simulink model "c00019M_harness"  (R2018a)
settings: Solver=ode3  StartTime=0.0  StopTime=10.0  RelTol=1e-3  EnableMultiTasking=on
undefined symbols (not defined in the file): b, DiscIntNeverNeededParam, J, K, L, PosMinimaW4, R, sigbuilder_block
(part 3 of 43)

== system c00019M_harness/Eval14 ==
  In1 : Inport
  In2 : Inport  Port=2
  In4 : Inport  Port=3
  Constant3 : Constant
  Data Type Conversion : DataTypeConversion
  Data Type Conversion1 : DataTypeConversion
  Data Type Conversion3 : DataTypeConversion
  Memory1 : Memory  InitialCondition=1
  Memory2 : Memory  InitialCondition=1
  Memory4 : Memory  InitialCondition=1
  MinMax : MinMax  Inputs=4
  MinMax1 : MinMax  Inputs=2
  MinMax2 : MinMax  Inputs=2
  MinMax4 : MinMax  Inputs=2
  ROOut1 : RelationalOperator  Operator===  OutDataTypeStr=boolean  RndMeth=Simplest
  ROOut2 : RelationalOperator  Operator===  OutDataTypeStr=boolean  RndMeth=Simplest
  ROOut4 : RelationalOperator  Operator===  OutDataTypeStr=boolean  RndMeth=Simplest
  Out1 : Outport
  wires:
  Data Type Conversion3/1 -> MinMax4/1
  Data Type Conversion1/1 -> MinMax2/1
  Data Type Conversion/1 -> MinMax1/1
  MinMax1/1 -> Memory1/1, MinMax/1
  ROOut4/1 -> Data Type Conversion3/1
  MinMax2/1 -> Memory2/1, MinMax/2
  ROOut1/1 -> Data Type Conversion/1
  Memory2/1 -> MinMax2/2
  Memory4/1 -> MinMax4/2
  ROOut2/1 -> Data Type Conversion1/1
  MinMax4/1 -> Memory4/1, MinMax/4
  Memory1/1 -> MinMax1/2
  [out4] -> ROOut4/2
  In4/1 -> ROOut4/1
  [out2] -> ROOut2/2
  In1/1 -> ROOut1/1
  In2/1 -> ROOut2/1
  [out1] -> ROOut1/2
  MinMax/1 -> Out1/1
  Constant3/1 -> MinMax/3

== system c00019M_harness/Eval141 ==
  In1 : Inport
  In2 : Inport  Port=2
  In4 : Inport  Port=3
  Constant3 : Constant
  Data Type Conversion : DataTypeConversion
  Data Type Conversion1 : DataTypeConversion
  Data Type Conversion3 : DataTypeConversion
  Memory1 : Memory  InitialCondition=1
  Memory2 : Memory  InitialCondition=1
  Memory4 : Memory  InitialCondition=1
  MinMax : MinMax  Inputs=4
  MinMax1 : MinMax  Inputs=2
  MinMax2 : MinMax  Inputs=2
  MinMax4 : MinMax  Inputs=2
  ROOut1 : RelationalOperator  Operator===  OutDataTypeStr=boolean  RndMeth=Simplest
  ROOut2 : RelationalOperator  Operator===  OutDataTypeStr=boolean  RndMeth=Simplest
  ROOut4 : RelationalOperator  Operator===  OutDataTypeStr=boolean  RndMeth=Simplest
  Out1 : Outport
  wires:
  Data Type Conversion3/1 -> MinMax4/1
  Data Type Conversion1/1 -> MinMax2/1
  Data Type Conversion/1 -> MinMax1/1
  MinMax1/1 -> Memory1/1, MinMax/1
  ROOut4/1 -> Data Type Conversion3/1
  MinMax2/1 -> Memory2/1, MinMax/2
  ROOut1/1 -> Data Type Conversion/1
  Memory2/1 -> MinMax2/2
  Memory4/1 -> MinMax4/2
  ROOut2/1 -> Data Type Conversion1/1
  MinMax4/1 -> Memory4/1, MinMax/4
  Memory1/1 -> MinMax1/2
  [out4] -> ROOut4/2
  In4/1 -> ROOut4/1
  [out2] -> ROOut2/2
  In1/1 -> ROOut1/1
  In2/1 -> ROOut2/1
  [out1] -> ROOut1/2
  MinMax/1 -> Out1/1
  Constant3/1 -> MinMax/3

== system c00019M_harness/Eval142 ==
  In1 : Inport
  In2 : Inport  Port=2
  In4 : Inport  Port=3
  Constant3 : Constant
  Data Type Conversion : DataTypeConversion
  Data Type Conversion1 : DataTypeConversion
  Data Type Conversion3 : DataTypeConversion
  Memory1 : Memory  InitialCondition=1
  Memory2 : Memory  InitialCondition=1
  Memory4 : Memory  InitialCondition=1
  MinMax : MinMax  Inputs=4
  MinMax1 : MinMax  Inputs=2
  MinMax2 : MinMax  Inputs=2
  MinMax4 : MinMax  Inputs=2
  ROOut1 : RelationalOperator  Operator===  OutDataTypeStr=boolean  RndMeth=Simplest
  ROOut2 : RelationalOperator  Operator===  OutDataTypeStr=boolean  RndMeth=Simplest
  ROOut4 : RelationalOperator  Operator===  OutDataTypeStr=boolean  RndMeth=Simplest
  Out1 : Outport
  wires:
  Data Type Conversion3/1 -> MinMax4/1
  Data Type Conversion1/1 -> MinMax2/1
  Data Type Conversion/1 -> MinMax1/1
  MinMax1/1 -> Memory1/1, MinMax/1
  ROOut4/1 -> Data Type Conversion3/1
  MinMax2/1 -> Memory2/1, MinMax/2
  ROOut1/1 -> Data Type Conversion/1
  Memory2/1 -> MinMax2/2
  Memory4/1 -> MinMax4/2
  ROOut2/1 -> Data Type Conversion1/1
  MinMax4/1 -> Memory4/1, MinMax/4
  Memory1/1 -> MinMax1/2
  [out4] -> ROOut4/2
  In4/1 -> ROOut4/1
  [out2] -> ROOut2/2
  In1/1 -> ROOut1/1
  In2/1 -> ROOut2/1
  [out1] -> ROOut1/2
  MinMax/1 -> Out1/1
  Constant3/1 -> MinMax/3

== system c00019M_harness/Eval143 ==
  In1 : Inport
  In2 : Inport  Port=2
  In4 : Inport  Port=3
  Constant3 : Constant
  Data Type Conversion : DataTypeConversion
  Data Type Conversion1 : DataTypeConversion
  Data Type Conversion3 : DataTypeConversion
  Memory1 : Memory  InitialCondition=1
  Memory2 : Memory  InitialCondition=1
  Memory4 : Memory  InitialCondition=1
  MinMax : MinMax  Inputs=4
  MinMax1 : MinMax  Inputs=2
  MinMax2 : MinMax  Inputs=2
  MinMax4 : MinMax  Inputs=2
  ROOut1 : RelationalOperator  Operator===  OutDataTypeStr=boolean  RndMeth=Simplest
  ROOut2 : RelationalOperator  Operator===  OutDataTypeStr=boolean  RndMeth=Simplest
  ROOut4 : RelationalOperator  Operator===  OutDataTypeStr=boolean  RndMeth=Simplest
  Out1 : Outport
  wires:
  Data Type Conversion3/1 -> MinMax4/1
  Data Type Conversion1/1 -> MinMax2/1
  Data Type Conversion/1 -> MinMax1/1
  MinMax1/1 -> Memory1/1, MinMax/1
  ROOut4/1 -> Data Type Conversion3/1
  MinMax2/1 -> Memory2/1, MinMax/2
  ROOut1/1 -> Data Type Conversion/1
  Memory2/1 -> MinMax2/2
  Memory4/1 -> MinMax4/2
  ROOut2/1 -> Data Type Conversion1/1
  MinMax4/1 -> Memory4/1, MinMax/4
  Memory1/1 -> MinMax1/2
  [out4] -> ROOut4/2
  In4/1 -> ROOut4/1
  [out2] -> ROOut2/2
  In1/1 -> ROOut1/1
  In2/1 -> ROOut2/1
  [out1] -> ROOut1/2
  MinMax/1 -> Out1/1
  Constant3/1 -> MinMax/3

== system c00019M_harness/Eval145 ==
  In1 : Inport
  In2 : Inport  Port=2
  In4 : Inport  Port=3
  Constant3 : Constant
  Data Type Conversion : DataTypeConversion
  Data Type Conversion1 : DataTypeConversion
  Data Type Conversion3 : DataTypeConversion
  Memory1 : Memory  InitialCondition=1
  Memory2 : Memory  InitialCondition=1
  Memory4 : Memory  InitialCondition=1
  MinMax : MinMax  Inputs=4
  MinMax1 : MinMax  Inputs=2
  MinMax2 : MinMax  Inputs=2
  MinMax4 : MinMax  Inputs=2
  ROOut1 : RelationalOperator  Operator===  OutDataTypeStr=boolean  RndMeth=Simplest
  ROOut2 : RelationalOperator  Operator===  OutDataTypeStr=boolean  RndMeth=Simplest
  ROOut4 : RelationalOperator  Operator===  OutDataTypeStr=boolean  RndMeth=Simplest
  Out1 : Outport
  wires:
  Data Type Conversion3/1 -> MinMax4/1
  Data Type Conversion1/1 -> MinMax2/1
  Data Type Conversion/1 -> MinMax1/1
  MinMax1/1 -> Memory1/1, MinMax/1
  ROOut4/1 -> Data Type Conversion3/1
  MinMax2/1 -> Memory2/1, MinMax/2
  ROOut1/1 -> Data Type Conversion/1
  Memory2/1 -> MinMax2/2
  Memory4/1 -> MinMax4/2
  ROOut2/1 -> Data Type Conversion1/1
  MinMax4/1 -> Memory4/1, MinMax/4
  Memory1/1 -> MinMax1/2
  [out4] -> ROOut4/2
  In4/1 -> ROOut4/1
  [out2] -> ROOut2/2
  In1/1 -> ROOut1/1
  In2/1 -> ROOut2/1
  [out1] -> ROOut1/2
  MinMax/1 -> Out1/1
  Constant3/1 -> MinMax/3

== system c00019M_harness/Eval146 ==
  In1 : Inport
  In2 : Inport  Port=2
  In4 : Inport  Port=3
  Constant3 : Constant
  Data Type Conversion : DataTypeConversion
  Data Type Conversion1 : DataTypeConversion
  Data Type Conversion3 : DataTypeConversion
  Memory1 : Memory  InitialCondition=1
  Memory2 : Memory  InitialCondition=1
  Memory4 : Memory  InitialCondition=1
  MinMax : MinMax  Inputs=4
  MinMax1 : MinMax  Inputs=2
  MinMax2 : MinMax  Inputs=2
  MinMax4 : MinMax  Inputs=2
  ROOut1 : RelationalOperator  Operator===  OutDataTypeStr=boolean  RndMeth=Simplest
  ROOut2 : RelationalOperator  Operator===  OutDataTypeStr=boolean  RndMeth=Simplest
  ROOut4 : RelationalOperator  Operator===  OutDataTypeStr=boolean  RndMeth=Simplest
  Out1 : Outport
  wires:
  Data Type Conversion3/1 -> MinMax4/1
  Data Type Conversion1/1 -> MinMax2/1
  Data Type Conversion/1 -> MinMax1/1
  MinMax1/1 -> Memory1/1, MinMax/1
  ROOut4/1 -> Data Type Conversion3/1
  MinMax2/1 -> Memory2/1, MinMax/2
  ROOut1/1 -> Data Type Conversion/1
  Memory2/1 -> MinMax2/2
  Memory4/1 -> MinMax4/2
  ROOut2/1 -> Data Type Conversion1/1
  MinMax4/1 -> Memory4/1, MinMax/4
  Memory1/1 -> MinMax1/2
  [out4] -> ROOut4/2
  In4/1 -> ROOut4/1
  [out2] -> ROOut2/2
  In1/1 -> ROOut1/1
  In2/1 -> ROOut2/1
  [out1] -> ROOut1/2
  MinMax/1 -> Out1/1
  Constant3/1 -> MinMax/3

== system c00019M_harness/Eval147 ==
  In1 : Inport
  In2 : Inport  Port=2
  In4 : Inport  Port=3
  Constant3 : Constant
  Data Type Conversion : DataTypeConversion
  Data Type Conversion1 : DataTypeConversion
  Data Type Conversion3 : DataTypeConversion
  Memory1 : Memory  InitialCondition=1
  Memory2 : Memory  InitialCondition=1
  Memory4 : Memory  InitialCondition=1
  MinMax : MinMax  Inputs=4
  MinMax1 : MinMax  Inputs=2
  MinMax2 : MinMax  Inputs=2
  MinMax4 : MinMax  Inputs=2
  ROOut1 : RelationalOperator  Operator===  OutDataTypeStr=boolean  RndMeth=Simplest
  ROOut2 : RelationalOperator  Operator===  OutDataTypeStr=boolean  RndMeth=Simplest
  ROOut4 : RelationalOperator  Operator===  OutDataTypeStr=boolean  RndMeth=Simplest
  Out1 : Outport
  wires:
  Data Type Conversion3/1 -> MinMax4/1
  Data Type Conversion1/1 -> MinMax2/1
  Data Type Conversion/1 -> MinMax1/1
  MinMax1/1 -> Memory1/1, MinMax/1
  ROOut4/1 -> Data Type Conversion3/1
  MinMax2/1 -> Memory2/1, MinMax/2
  ROOut1/1 -> Data Type Conversion/1
  Memory2/1 -> MinMax2/2
  Memory4/1 -> MinMax4/2
  ROOut2/1 -> Data Type Conversion1/1
  MinMax4/1 -> Memory4/1, MinMax/4
  Memory1/1 -> MinMax1/2
  [out4] -> ROOut4/2
  In4/1 -> ROOut4/1
  [out2] -> ROOut2/2
  In1/1 -> ROOut1/1
  In2/1 -> ROOut2/1
  [out1] -> ROOut1/2
  MinMax/1 -> Out1/1
  Constant3/1 -> MinMax/3

== system c00019M_harness/Eval149 ==
  In1 : Inport
  In2 : Inport  Port=2
  In4 : Inport  Port=3
  Constant3 : Constant
  Data Type Conversion : DataTypeConversion
  Data Type Conversion1 : DataTypeConversion
  Data Type Conversion3 : DataTypeConversion
  Memory1 : Memory  InitialCondition=1
  Memory2 : Memory  InitialCondition=1
  Memory4 : Memory  InitialCondition=1
  MinMax : MinMax  Inputs=4
  MinMax1 : MinMax  Inputs=2
  MinMax2 : MinMax  Inputs=2
  MinMax4 : MinMax  Inputs=2
  ROOut1 : RelationalOperator  Operator===  OutDataTypeStr=boolean  RndMeth=Simplest
  ROOut2 : RelationalOperator  Operator===  OutDataTypeStr=boolean  RndMeth=Simplest
  ROOut4 : RelationalOperator  Operator===  OutDataTypeStr=boolean  RndMeth=Simplest
  Out1 : Outport
  wires:
  Data Type Conversion3/1 -> MinMax4/1
  Data Type Conversion1/1 -> MinMax2/1
  Data Type Conversion/1 -> MinMax1/1
  MinMax1/1 -> Memory1/1, MinMax/1
  ROOut4/1 -> Data Type Conversion3/1
  MinMax2/1 -> Memory2/1, MinMax/2
  ROOut1/1 -> Data Type Conversion/1
  Memory2/1 -> MinMax2/2
  Memory4/1 -> MinMax4/2
  ROOut2/1 -> Data Type Conversion1/1
  MinMax4/1 -> Memory4/1, MinMax/4
  Memory1/1 -> MinMax1/2
  [out4] -> ROOut4/2
  In4/1 -> ROOut4/1
  [out2] -> ROOut2/2
  In1/1 -> ROOut1/1
  In2/1 -> ROOut2/1
  [out1] -> ROOut1/2
  MinMax/1 -> Out1/1
  Constant3/1 -> MinMax/3

== system c00019M_harness/Eval15 ==
  In1 : Inport
  In2 : Inport  Port=2
  In4 : Inport  Port=3
  Constant3 : Constant
  Data Type Conversion : DataTypeConversion
  Data Type Conversion1 : DataTypeConversion
  Data Type Conversion3 : DataTypeConversion
  Memory1 : Memory  InitialCondition=1
  Memory2 : Memory  InitialCondition=1
  Memory4 : Memory  InitialCondition=1
  MinMax : MinMax  Inputs=4
  MinMax1 : MinMax  Inputs=2
  MinMax2 : MinMax  Inputs=2
  MinMax4 : MinMax  Inputs=2
  ROOut1 : RelationalOperator  Operator===  OutDataTypeStr=boolean  RndMeth=Simplest
  ROOut2 : RelationalOperator  Operator===  OutDataTypeStr=boolean  RndMeth=Simplest
  ROOut4 : RelationalOperator  Operator===  OutDataTypeStr=boolean  RndMeth=Simplest
  Out1 : Outport
  wires:
  Data Type Conversion3/1 -> MinMax4/1
  Data Type Conversion1/1 -> MinMax2/1
  Data Type Conversion/1 -> MinMax1/1
  MinMax1/1 -> Memory1/1, MinMax/1
  ROOut4/1 -> Data Type Conversion3/1
  MinMax2/1 -> Memory2/1, MinMax/2
  ROOut1/1 -> Data Type Conversion/1
  Memory2/1 -> MinMax2/2
  Memory4/1 -> MinMax4/2
  ROOut2/1 -> Data Type Conversion1/1
  MinMax4/1 -> Memory4/1, MinMax/4
  Memory1/1 -> MinMax1/2
  [out4] -> ROOut4/2
  In4/1 -> ROOut4/1
  [out2] -> ROOut2/2
  In1/1 -> ROOut1/1
  In2/1 -> ROOut2/1
  [out1] -> ROOut1/2
  MinMax/1 -> Out1/1
  Constant3/1 -> MinMax/3

== system c00019M_harness/Eval150 ==
  In1 : Inport
  In2 : Inport  Port=2
  In4 : Inport  Port=3
  Constant3 : Constant
  Data Type Conversion : DataTypeConversion
  Data Type Conversion1 : DataTypeConversion
  Data Type Conversion3 : DataTypeConversion
  Memory1 : Memory  InitialCondition=1
  Memory2 : Memory  InitialCondition=1
  Memory4 : Memory  InitialCondition=1
  MinMax : MinMax  Inputs=4
  MinMax1 : MinMax  Inputs=2
  MinMax2 : MinMax  Inputs=2
  MinMax4 : MinMax  Inputs=2
  ROOut1 : RelationalOperator  Operator===  OutDataTypeStr=boolean  RndMeth=Simplest
  ROOut2 : RelationalOperator  Operator===  OutDataTypeStr=boolean  RndMeth=Simplest
  ROOut4 : RelationalOperator  Operator===  OutDataTypeStr=boolean  RndMeth=Simplest
  Out1 : Outport
  wires:
  Data Type Conversion3/1 -> MinMax4/1
  Data Type Conversion1/1 -> MinMax2/1
  Data Type Conversion/1 -> MinMax1/1
  MinMax1/1 -> Memory1/1, MinMax/1
  ROOut4/1 -> Data Type Conversion3/1
  MinMax2/1 -> Memory2/1, MinMax/2
  ROOut1/1 -> Data Type Conversion/1
  Memory2/1 -> MinMax2/2
  Memory4/1 -> MinMax4/2
  ROOut2/1 -> Data Type Conversion1/1
  MinMax4/1 -> Memory4/1, MinMax/4
  Memory1/1 -> MinMax1/2
  [out4] -> ROOut4/2
  In4/1 -> ROOut4/1
  [out2] -> ROOut2/2
  In1/1 -> ROOut1/1
  In2/1 -> ROOut2/1
  [out1] -> ROOut1/2
  MinMax/1 -> Out1/1
  Constant3/1 -> MinMax/3

== system c00019M_harness/Eval151 ==
  In1 : Inport
  In2 : Inport  Port=2
  In4 : Inport  Port=3
  Constant3 : Constant
  Data Type Conversion : DataTypeConversion
  Data Type Conversion1 : DataTypeConversion
  Data Type Conversion3 : DataTypeConversion
  Memory1 : Memory  InitialCondition=1
  Memory2 : Memory  InitialCondition=1
  Memory4 : Memory  InitialCondition=1
  MinMax : MinMax  Inputs=4
  MinMax1 : MinMax  Inputs=2
  MinMax2 : MinMax  Inputs=2
  MinMax4 : MinMax  Inputs=2
  ROOut1 : RelationalOperator  Operator===  OutDataTypeStr=boolean  RndMeth=Simplest
  ROOut2 : RelationalOperator  Operator===  OutDataTypeStr=boolean  RndMeth=Simplest
  ROOut4 : RelationalOperator  Operator===  OutDataTypeStr=boolean  RndMeth=Simplest
  Out1 : Outport
  wires:
  Data Type Conversion3/1 -> MinMax4/1
  Data Type Conversion1/1 -> MinMax2/1
  Data Type Conversion/1 -> MinMax1/1
  MinMax1/1 -> Memory1/1, MinMax/1
  ROOut4/1 -> Data Type Conversion3/1
  MinMax2/1 -> Memory2/1, MinMax/2
  ROOut1/1 -> Data Type Conversion/1
  Memory2/1 -> MinMax2/2
  Memory4/1 -> MinMax4/2
  ROOut2/1 -> Data Type Conversion1/1
  MinMax4/1 -> Memory4/1, MinMax/4
  Memory1/1 -> MinMax1/2
  [out4] -> ROOut4/2
  In4/1 -> ROOut4/1
  [out2] -> ROOut2/2
  In1/1 -> ROOut1/1
  In2/1 -> ROOut2/1
  [out1] -> ROOut1/2
  MinMax/1 -> Out1/1
  Constant3/1 -> MinMax/3

== system c00019M_harness/Eval153 ==
  In1 : Inport
  In2 : Inport  Port=2
  In4 : Inport  Port=3
  Constant3 : Constant
  Data Type Conversion : DataTypeConversion
  Data Type Conversion1 : DataTypeConversion
  Data Type Conversion3 : DataTypeConversion
  Memory1 : Memory  InitialCondition=1
  Memory2 : Memory  InitialCondition=1
  Memory4 : Memory  InitialCondition=1
  MinMax : MinMax  Inputs=4
  MinMax1 : MinMax  Inputs=2
  MinMax2 : MinMax  Inputs=2
  MinMax4 : MinMax  Inputs=2
  ROOut1 : RelationalOperator  Operator===  OutDataTypeStr=boolean  RndMeth=Simplest
  ROOut2 : RelationalOperator  Operator===  OutDataTypeStr=boolean  RndMeth=Simplest
  ROOut4 : RelationalOperator  Operator===  OutDataTypeStr=boolean  RndMeth=Simplest
  Out1 : Outport
  wires:
  Data Type Conversion3/1 -> MinMax4/1
  Data Type Conversion1/1 -> MinMax2/1
  Data Type Conversion/1 -> MinMax1/1
  MinMax1/1 -> Memory1/1, MinMax/1
  ROOut4/1 -> Data Type Conversion3/1
  MinMax2/1 -> Memory2/1, MinMax/2
  ROOut1/1 -> Data Type Conversion/1
  Memory2/1 -> MinMax2/2
  Memory4/1 -> MinMax4/2
  ROOut2/1 -> Data Type Conversion1/1
  MinMax4/1 -> Memory4/1, MinMax/4
  Memory1/1 -> MinMax1/2
  [out4] -> ROOut4/2
  In4/1 -> ROOut4/1
  [out2] -> ROOut2/2
  In1/1 -> ROOut1/1
  In2/1 -> ROOut2/1
  [out1] -> ROOut1/2
  MinMax/1 -> Out1/1
  Constant3/1 -> MinMax/3

== system c00019M_harness/Eval154 ==
  In1 : Inport
  In2 : Inport  Port=2
  In4 : Inport  Port=3
  Constant3 : Constant
  Data Type Conversion : DataTypeConversion
  Data Type Conversion1 : DataTypeConversion
  Data Type Conversion3 : DataTypeConversion
  Memory1 : Memory  InitialCondition=1
  Memory2 : Memory  InitialCondition=1
  Memory4 : Memory  InitialCondition=1
  MinMax : MinMax  Inputs=4
  MinMax1 : MinMax  Inputs=2
  MinMax2 : MinMax  Inputs=2
  MinMax4 : MinMax  Inputs=2
  ROOut1 : RelationalOperator  Operator===  OutDataTypeStr=boolean  RndMeth=Simplest
  ROOut2 : RelationalOperator  Operator===  OutDataTypeStr=boolean  RndMeth=Simplest
  ROOut4 : RelationalOperator  Operator===  OutDataTypeStr=boolean  RndMeth=Simplest
  Out1 : Outport
  wires:
  Data Type Conversion3/1 -> MinMax4/1
  Data Type Conversion1/1 -> MinMax2/1
  Data Type Conversion/1 -> MinMax1/1
  MinMax1/1 -> Memory1/1, MinMax/1
  ROOut4/1 -> Data Type Conversion3/1
  MinMax2/1 -> Memory2/1, MinMax/2
  ROOut1/1 -> Data Type Conversion/1
  Memory2/1 -> MinMax2/2
  Memory4/1 -> MinMax4/2
  ROOut2/1 -> Data Type Conversion1/1
  MinMax4/1 -> Memory4/1, MinMax/4
  Memory1/1 -> MinMax1/2
  [out4] -> ROOut4/2
  In4/1 -> ROOut4/1
  [out2] -> ROOut2/2
  In1/1 -> ROOut1/1
  In2/1 -> ROOut2/1
  [out1] -> ROOut1/2
  MinMax/1 -> Out1/1
  Constant3/1 -> MinMax/3

== system c00019M_harness/Eval155 ==
  In1 : Inport
  In2 : Inport  Port=2
  In4 : Inport  Port=3
  Constant3 : Constant
  Data Type Conversion : DataTypeConversion
  Data Type Conversion1 : DataTypeConversion
  Data Type Conversion3 : DataTypeConversion
  Memory1 : Memory  InitialCondition=1
  Memory2 : Memory  InitialCondition=1
  Memory4 : Memory  InitialCondition=1
  MinMax : MinMax  Inputs=4
  MinMax1 : MinMax  Inputs=2
  MinMax2 : MinMax  Inputs=2
  MinMax4 : MinMax  Inputs=2
  ROOut1 : RelationalOperator  Operator===  OutDataTypeStr=boolean  RndMeth=Simplest
  ROOut2 : RelationalOperator  Operator===  OutDataTypeStr=boolean  RndMeth=Simplest
  ROOut4 : RelationalOperator  Operator===  OutDataTypeStr=boolean  RndMeth=Simplest
  Out1 : Outport
  wires:
  Data Type Conversion3/1 -> MinMax4/1
  Data Type Conversion1/1 -> MinMax2/1
  Data Type Conversion/1 -> MinMax1/1
  MinMax1/1 -> Memory1/1, MinMax/1
  ROOut4/1 -> Data Type Conversion3/1
  MinMax2/1 -> Memory2/1, MinMax/2
  ROOut1/1 -> Data Type Conversion/1
  Memory2/1 -> MinMax2/2
  Memory4/1 -> MinMax4/2
  ROOut2/1 -> Data Type Conversion1/1
  MinMax4/1 -> Memory4/1, MinMax/4
  Memory1/1 -> MinMax1/2
  [out4] -> ROOut4/2
  In4/1 -> ROOut4/1
  [out2] -> ROOut2/2
  In1/1 -> ROOut1/1
  In2/1 -> ROOut2/1
  [out1] -> ROOut1/2
  MinMax/1 -> Out1/1
  Constant3/1 -> MinMax/3

== system c00019M_harness/Eval157 ==
  In1 : Inport
  In2 : Inport  Port=2
  In4 : Inport  Port=3
  Constant3 : Constant
  Data Type Conversion : DataTypeConversion
  Data Type Conversion1 : DataTypeConversion
  Data Type Conversion3 : DataTypeConversion
  Memory1 : Memory  InitialCondition=1
  Memory2 : Memory  InitialCondition=1
  Memory4 : Memory  InitialCondition=1
  MinMax : MinMax  Inputs=4
  MinMax1 : MinMax  Inputs=2
  MinMax2 : MinMax  Inputs=2
  MinMax4 : MinMax  Inputs=2
  ROOut1 : RelationalOperator  Operator===  OutDataTypeStr=boolean  RndMeth=Simplest
  ROOut2 : RelationalOperator  Operator===  OutDataTypeStr=boolean  RndMeth=Simplest
  ROOut4 : RelationalOperator  Operator===  OutDataTypeStr=boolean  RndMeth=Simplest
  Out1 : Outport
  wires:
  Data Type Conversion3/1 -> MinMax4/1
  Data Type Conversion1/1 -> MinMax2/1
  Data Type Conversion/1 -> MinMax1/1
  MinMax1/1 -> Memory1/1, MinMax/1
  ROOut4/1 -> Data Type Conversion3/1
  MinMax2/1 -> Memory2/1, MinMax/2
  ROOut1/1 -> Data Type Conversion/1
  Memory2/1 -> MinMax2/2
  Memory4/1 -> MinMax4/2
  ROOut2/1 -> Data Type Conversion1/1
  MinMax4/1 -> Memory4/1, MinMax/4
  Memory1/1 -> MinMax1/2
  [out4] -> ROOut4/2
  In4/1 -> ROOut4/1
  [out2] -> ROOut2/2
  In1/1 -> ROOut1/1
  In2/1 -> ROOut2/1
  [out1] -> ROOut1/2
  MinMax/1 -> Out1/1
  Constant3/1 -> MinMax/3

== system c00019M_harness/Eval158 ==
  In1 : Inport
  In2 : Inport  Port=2
  In4 : Inport  Port=3
  Constant3 : Constant
  Data Type Conversion : DataTypeConversion
  Data Type Conversion1 : DataTypeConversion
  Data Type Conversion3 : DataTypeConversion
  Memory1 : Memory  InitialCondition=1
  Memory2 : Memory  InitialCondition=1
  Memory4 : Memory  InitialCondition=1
  MinMax : MinMax  Inputs=4
  MinMax1 : MinMax  Inputs=2
  MinMax2 : MinMax  Inputs=2
  MinMax4 : MinMax  Inputs=2
  ROOut1 : RelationalOperator  Operator===  OutDataTypeStr=boolean  RndMeth=Simplest
  ROOut2 : RelationalOperator  Operator===  OutDataTypeStr=boolean  RndMeth=Simplest
  ROOut4 : RelationalOperator  Operator===  OutDataTypeStr=boolean  RndMeth=Simplest
  Out1 : Outport
  wires:
  Data Type Conversion3/1 -> MinMax4/1
  Data Type Conversion1/1 -> MinMax2/1
  Data Type Conversion/1 -> MinMax1/1
  MinMax1/1 -> Memory1/1, MinMax/1
  ROOut4/1 -> Data Type Conversion3/1
  MinMax2/1 -> Memory2/1, MinMax/2
  ROOut1/1 -> Data Type Conversion/1
  Memory2/1 -> MinMax2/2
  Memory4/1 -> MinMax4/2
  ROOut2/1 -> Data Type Conversion1/1
  MinMax4/1 -> Memory4/1, MinMax/4
  Memory1/1 -> MinMax1/2
  [out4] -> ROOut4/2
  In4/1 -> ROOut4/1
  [out2] -> ROOut2/2
  In1/1 -> ROOut1/1
  In2/1 -> ROOut2/1
  [out1] -> ROOut1/2
  MinMax/1 -> Out1/1
  Constant3/1 -> MinMax/3

== system c00019M_harness/Eval159 ==
  In1 : Inport
  In2 : Inport  Port=2
  In4 : Inport  Port=3
  Constant3 : Constant
  Data Type Conversion : DataTypeConversion
  Data Type Conversion1 : DataTypeConversion
  Data Type Conversion3 : DataTypeConversion
  Memory1 : Memory  InitialCondition=1
  Memory2 : Memory  InitialCondition=1
  Memory4 : Memory  InitialCondition=1
  MinMax : MinMax  Inputs=4
  MinMax1 : MinMax  Inputs=2
  MinMax2 : MinMax  Inputs=2
  MinMax4 : MinMax  Inputs=2
  ROOut1 : RelationalOperator  Operator===  OutDataTypeStr=boolean  RndMeth=Simplest
  ROOut2 : RelationalOperator  Operator===  OutDataTypeStr=boolean  RndMeth=Simplest
  ROOut4 : RelationalOperator  Operator===  OutDataTypeStr=boolean  RndMeth=Simplest
  Out1 : Outport
  wires:
  Data Type Conversion3/1 -> MinMax4/1
  Data Type Conversion1/1 -> MinMax2/1
  Data Type Conversion/1 -> MinMax1/1
  MinMax1/1 -> Memory1/1, MinMax/1
  ROOut4/1 -> Data Type Conversion3/1
  MinMax2/1 -> Memory2/1, MinMax/2
  ROOut1/1 -> Data Type Conversion/1
  Memory2/1 -> MinMax2/2
  Memory4/1 -> MinMax4/2
  ROOut2/1 -> Data Type Conversion1/1
  MinMax4/1 -> Memory4/1, MinMax/4
  Memory1/1 -> MinMax1/2
  [out4] -> ROOut4/2
  In4/1 -> ROOut4/1
  [out2] -> ROOut2/2
  In1/1 -> ROOut1/1
  In2/1 -> ROOut2/1
  [out1] -> ROOut1/2
  MinMax/1 -> Out1/1
  Constant3/1 -> MinMax/3

== system c00019M_harness/Eval161 ==
  In1 : Inport
  In2 : Inport  Port=2
  In4 : Inport  Port=3
  Constant3 : Constant
  Data Type Conversion : DataTypeConversion
  Data Type Conversion1 : DataTypeConversion
  Data Type Conversion3 : DataTypeConversion
  Memory1 : Memory  InitialCondition=1
  Memory2 : Memory  InitialCondition=1
  Memory4 : Memory  InitialCondition=1
  MinMax : MinMax  Inputs=4
  MinMax1 : MinMax  Inputs=2
  MinMax2 : MinMax  Inputs=2
  MinMax4 : MinMax  Inputs=2
  ROOut1 : RelationalOperator  Operator===  OutDataTypeStr=boolean  RndMeth=Simplest
  ROOut2 : RelationalOperator  Operator===  OutDataTypeStr=boolean  RndMeth=Simplest
  ROOut4 : RelationalOperator  Operator===  OutDataTypeStr=boolean  RndMeth=Simplest
  Out1 : Outport
  wires:
  Data Type Conversion3/1 -> MinMax4/1
  Data Type Conversion1/1 -> MinMax2/1
  Data Type Conversion/1 -> MinMax1/1
  MinMax1/1 -> Memory1/1, MinMax/1
  ROOut4/1 -> Data Type Conversion3/1
  MinMax2/1 -> Memory2/1, MinMax/2
  ROOut1/1 -> Data Type Conversion/1
  Memory2/1 -> MinMax2/2
  Memory4/1 -> MinMax4/2
  ROOut2/1 -> Data Type Conversion1/1
  MinMax4/1 -> Memory4/1, MinMax/4
  Memory1/1 -> MinMax1/2
  [out4] -> ROOut4/2
  In4/1 -> ROOut4/1
  [out2] -> ROOut2/2
  In1/1 -> ROOut1/1
  In2/1 -> ROOut2/1
  [out1] -> ROOut1/2
  MinMax/1 -> Out1/1
  Constant3/1 -> MinMax/3

== system c00019M_harness/Eval162 ==
  In1 : Inport
  In2 : Inport  Port=2
  In4 : Inport  Port=3
  Constant3 : Constant
  Data Type Conversion : DataTypeConversion
  Data Type Conversion1 : DataTypeConversion
  Data Type Conversion3 : DataTypeConversion
  Memory1 : Memory  InitialCondition=1
  Memory2 : Memory  InitialCondition=1
  Memory4 : Memory  InitialCondition=1
  MinMax : MinMax  Inputs=4
  MinMax1 : MinMax  Inputs=2
  MinMax2 : MinMax  Inputs=2
  MinMax4 : MinMax  Inputs=2
  ROOut1 : RelationalOperator  Operator===  OutDataTypeStr=boolean  RndMeth=Simplest
  ROOut2 : RelationalOperator  Operator===  OutDataTypeStr=boolean  RndMeth=Simplest
  ROOut4 : RelationalOperator  Operator===  OutDataTypeStr=boolean  RndMeth=Simplest
  Out1 : Outport
  wires:
  Data Type Conversion3/1 -> MinMax4/1
  Data Type Conversion1/1 -> MinMax2/1
  Data Type Conversion/1 -> MinMax1/1
  MinMax1/1 -> Memory1/1, MinMax/1
  ROOut4/1 -> Data Type Conversion3/1
  MinMax2/1 -> Memory2/1, MinMax/2
  ROOut1/1 -> Data Type Conversion/1
  Memory2/1 -> MinMax2/2
  Memory4/1 -> MinMax4/2
  ROOut2/1 -> Data Type Conversion1/1
  MinMax4/1 -> Memory4/1, MinMax/4
  Memory1/1 -> MinMax1/2
  [out4] -> ROOut4/2
  In4/1 -> ROOut4/1
  [out2] -> ROOut2/2
  In1/1 -> ROOut1/1
  In2/1 -> ROOut2/1
  [out1] -> ROOut1/2
  MinMax/1 -> Out1/1
  Constant3/1 -> MinMax/3

== system c00019M_harness/Eval163 ==
  In1 : Inport
  In2 : Inport  Port=2
  In4 : Inport  Port=3
  Constant3 : Constant
  Data Type Conversion : DataTypeConversion
  Data Type Conversion1 : DataTypeConversion
  Data Type Conversion3 : DataTypeConversion
  Memory1 : Memory  InitialCondition=1
  Memory2 : Memory  InitialCondition=1
  Memory4 : Memory  InitialCondition=1
  MinMax : MinMax  Inputs=4
  MinMax1 : MinMax  Inputs=2
  MinMax2 : MinMax  Inputs=2
  MinMax4 : MinMax  Inputs=2
  ROOut1 : RelationalOperator  Operator===  OutDataTypeStr=boolean  RndMeth=Simplest
  ROOut2 : RelationalOperator  Operator===  OutDataTypeStr=boolean  RndMeth=Simplest
  ROOut4 : RelationalOperator  Operator===  OutDataTypeStr=boolean  RndMeth=Simplest
  Out1 : Outport
  wires:
  Data Type Conversion3/1 -> MinMax4/1
  Data Type Conversion1/1 -> MinMax2/1
  Data Type Conversion/1 -> MinMax1/1
  MinMax1/1 -> Memory1/1, MinMax/1
  ROOut4/1 -> Data Type Conversion3/1
  MinMax2/1 -> Memory2/1, MinMax/2
  ROOut1/1 -> Data Type Conversion/1
  Memory2/1 -> MinMax2/2
  Memory4/1 -> MinMax4/2
  ROOut2/1 -> Data Type Conversion1/1
  MinMax4/1 -> Memory4/1, MinMax/4
  Memory1/1 -> MinMax1/2
  [out4] -> ROOut4/2
  In4/1 -> ROOut4/1
  [out2] -> ROOut2/2
  In1/1 -> ROOut1/1
  In2/1 -> ROOut2/1
  [out1] -> ROOut1/2
  MinMax/1 -> Out1/1
  Constant3/1 -> MinMax/3

== system c00019M_harness/Eval165 ==
  In1 : Inport
  In2 : Inport  Port=2
  In4 : Inport  Port=3
  Constant3 : Constant
  Data Type Conversion : DataTypeConversion
  Data Type Conversion1 : DataTypeConversion
  Data Type Conversion3 : DataTypeConversion
  Memory1 : Memory  InitialCondition=1
  Memory2 : Memory  InitialCondition=1
  Memory4 : Memory  InitialCondition=1
  MinMax : MinMax  Inputs=4
  MinMax1 : MinMax  Inputs=2
  MinMax2 : MinMax  Inputs=2
  MinMax4 : MinMax  Inputs=2
  ROOut1 : RelationalOperator  Operator===  OutDataTypeStr=boolean  RndMeth=Simplest
  ROOut2 : RelationalOperator  Operator===  OutDataTypeStr=boolean  RndMeth=Simplest
  ROOut4 : RelationalOperator  Operator===  OutDataTypeStr=boolean  RndMeth=Simplest
  Out1 : Outport
  wires:
  Data Type Conversion3/1 -> MinMax4/1
  Data Type Conversion1/1 -> MinMax2/1
  Data Type Conversion/1 -> MinMax1/1
  MinMax1/1 -> Memory1/1, MinMax/1
  ROOut4/1 -> Data Type Conversion3/1
  MinMax2/1 -> Memory2/1, MinMax/2
  ROOut1/1 -> Data Type Conversion/1
  Memory2/1 -> MinMax2/2
  Memory4/1 -> MinMax4/2
  ROOut2/1 -> Data Type Conversion1/1
  MinMax4/1 -> Memory4/1, MinMax/4
  Memory1/1 -> MinMax1/2
  [out4] -> ROOut4/2
  In4/1 -> ROOut4/1
  [out2] -> ROOut2/2
  In1/1 -> ROOut1/1
  In2/1 -> ROOut2/1
  [out1] -> ROOut1/2
  MinMax/1 -> Out1/1
  Constant3/1 -> MinMax/3

== system c00019M_harness/Eval166 ==
  In1 : Inport
  In2 : Inport  Port=2
  In4 : Inport  Port=3
  Constant3 : Constant
  Data Type Conversion : DataTypeConversion
  Data Type Conversion1 : DataTypeConversion
  Data Type Conversion3 : DataTypeConversion
  Memory1 : Memory  InitialCondition=1
  Memory2 : Memory  InitialCondition=1
  Memory4 : Memory  InitialCondition=1
  MinMax : MinMax  Inputs=4
  MinMax1 : MinMax  Inputs=2
  MinMax2 : MinMax  Inputs=2
  MinMax4 : MinMax  Inputs=2
  ROOut1 : RelationalOperator  Operator===  OutDataTypeStr=boolean  RndMeth=Simplest
  ROOut2 : RelationalOperator  Operator===  OutDataTypeStr=boolean  RndMeth=Simplest
  ROOut4 : RelationalOperator  Operator===  OutDataTypeStr=boolean  RndMeth=Simplest
  Out1 : Outport
  wires:
  Data Type Conversion3/1 -> MinMax4/1
  Data Type Conversion1/1 -> MinMax2/1
  Data Type Conversion/1 -> MinMax1/1
  MinMax1/1 -> Memory1/1, MinMax/1
  ROOut4/1 -> Data Type Conversion3/1
  MinMax2/1 -> Memory2/1, MinMax/2
  ROOut1/1 -> Data Type Conversion/1
  Memory2/1 -> MinMax2/2
  Memory4/1 -> MinMax4/2
  ROOut2/1 -> Data Type Conversion1/1
  MinMax4/1 -> Memory4/1, MinMax/4
  Memory1/1 -> MinMax1/2
  [out4] -> ROOut4/2
  In4/1 -> ROOut4/1
  [out2] -> ROOut2/2
  In1/1 -> ROOut1/1
  In2/1 -> ROOut2/1
  [out1] -> ROOut1/2
  MinMax/1 -> Out1/1
  Constant3/1 -> MinMax/3

== system c00019M_harness/Eval167 ==
  In1 : Inport
  In2 : Inport  Port=2
  In4 : Inport  Port=3
  Constant3 : Constant
  Data Type Conversion : DataTypeConversion
  Data Type Conversion1 : DataTypeConversion
  Data Type Conversion3 : DataTypeConversion
  Memory1 : Memory  InitialCondition=1
  Memory2 : Memory  InitialCondition=1
  Memory4 : Memory  InitialCondition=1
  MinMax : MinMax  Inputs=4
  MinMax1 : MinMax  Inputs=2
  MinMax2 : MinMax  Inputs=2
  MinMax4 : MinMax  Inputs=2
  ROOut1 : RelationalOperator  Operator===  OutDataTypeStr=boolean  RndMeth=Simplest
  ROOut2 : RelationalOperator  Operator===  OutDataTypeStr=boolean  RndMeth=Simplest
  ROOut4 : RelationalOperator  Operator===  OutDataTypeStr=boolean  RndMeth=Simplest
  Out1 : Outport
  wires:
  Data Type Conversion3/1 -> MinMax4/1
  Data Type Conversion1/1 -> MinMax2/1
  Data Type Conversion/1 -> MinMax1/1
  MinMax1/1 -> Memory1/1, MinMax/1
  ROOut4/1 -> Data Type Conversion3/1
  MinMax2/1 -> Memory2/1, MinMax/2
  ROOut1/1 -> Data Type Conversion/1
  Memory2/1 -> MinMax2/2
  Memory4/1 -> MinMax4/2
  ROOut2/1 -> Data Type Conversion1/1
  MinMax4/1 -> Memory4/1, MinMax/4
  Memory1/1 -> MinMax1/2
  [out4] -> ROOut4/2
  In4/1 -> ROOut4/1
  [out2] -> ROOut2/2
  In1/1 -> ROOut1/1
  In2/1 -> ROOut2/1
  [out1] -> ROOut1/2
  MinMax/1 -> Out1/1
  Constant3/1 -> MinMax/3

== system c00019M_harness/Eval169 ==
  In1 : Inport
  In2 : Inport  Port=2
  In4 : Inport  Port=3
  Constant3 : Constant
  Data Type Conversion : DataTypeConversion
  Data Type Conversion1 : DataTypeConversion
  Data Type Conversion3 : DataTypeConversion
  Memory1 : Memory  InitialCondition=1
  Memory2 : Memory  InitialCondition=1
  Memory4 : Memory  InitialCondition=1
  MinMax : MinMax  Inputs=4
  MinMax1 : MinMax  Inputs=2
  MinMax2 : MinMax  Inputs=2
  MinMax4 : MinMax  Inputs=2
  ROOut1 : RelationalOperator  Operator===  OutDataTypeStr=boolean  RndMeth=Simplest
  ROOut2 : RelationalOperator  Operator===  OutDataTypeStr=boolean  RndMeth=Simplest
  ROOut4 : RelationalOperator  Operator===  OutDataTypeStr=boolean  RndMeth=Simplest
  Out1 : Outport
  wires:
  Data Type Conversion3/1 -> MinMax4/1
  Data Type Conversion1/1 -> MinMax2/1
  Data Type Conversion/1 -> MinMax1/1
  MinMax1/1 -> Memory1/1, MinMax/1
  ROOut4/1 -> Data Type Conversion3/1
  MinMax2/1 -> Memory2/1, MinMax/2
  ROOut1/1 -> Data Type Conversion/1
  Memory2/1 -> MinMax2/2
  Memory4/1 -> MinMax4/2
  ROOut2/1 -> Data Type Conversion1/1
  MinMax4/1 -> Memory4/1, MinMax/4
  Memory1/1 -> MinMax1/2
  [out4] -> ROOut4/2
  In4/1 -> ROOut4/1
  [out2] -> ROOut2/2
  In1/1 -> ROOut1/1
  In2/1 -> ROOut2/1
  [out1] -> ROOut1/2
  MinMax/1 -> Out1/1
  Constant3/1 -> MinMax/3

== system c00019M_harness/Eval17 ==
  In1 : Inport
  In2 : Inport  Port=2
  In4 : Inport  Port=3
  Constant3 : Constant
  Data Type Conversion : DataTypeConversion
  Data Type Conversion1 : DataTypeConversion
  Data Type Conversion3 : DataTypeConversion
  Memory1 : Memory  InitialCondition=1
  Memory2 : Memory  InitialCondition=1
  Memory4 : Memory  InitialCondition=1
  MinMax : MinMax  Inputs=4
  MinMax1 : MinMax  Inputs=2
  MinMax2 : MinMax  Inputs=2
  MinMax4 : MinMax  Inputs=2
  ROOut1 : RelationalOperator  Operator===  OutDataTypeStr=boolean  RndMeth=Simplest
  ROOut2 : RelationalOperator  Operator===  OutDataTypeStr=boolean  RndMeth=Simplest
  ROOut4 : RelationalOperator  Operator===  OutDataTypeStr=boolean  RndMeth=Simplest
  Out1 : Outport
  wires:
  Data Type Conversion3/1 -> MinMax4/1
  Data Type Conversion1/1 -> MinMax2/1
  Data Type Conversion/1 -> MinMax1/1
  MinMax1/1 -> Memory1/1, MinMax/1
  ROOut4/1 -> Data Type Conversion3/1
  MinMax2/1 -> Memory2/1, MinMax/2
  ROOut1/1 -> Data Type Conversion/1
  Memory2/1 -> MinMax2/2
  Memory4/1 -> MinMax4/2
  ROOut2/1 -> Data Type Conversion1/1
  MinMax4/1 -> Memory4/1, MinMax/4
  Memory1/1 -> MinMax1/2
  [out4] -> ROOut4/2
  In4/1 -> ROOut4/1
  [out2] -> ROOut2/2
  In1/1 -> ROOut1/1
  In2/1 -> ROOut2/1
  [out1] -> ROOut1/2
  MinMax/1 -> Out1/1
  Constant3/1 -> MinMax/3

== system c00019M_harness/Eval170 ==
  In1 : Inport
  In2 : Inport  Port=2
  In4 : Inport  Port=3
  Constant3 : Constant
  Data Type Conversion : DataTypeConversion
  Data Type Conversion1 : DataTypeConversion
  Data Type Conversion3 : DataTypeConversion
  Memory1 : Memory  InitialCondition=1
  Memory2 : Memory  InitialCondition=1
  Memory4 : Memory  InitialCondition=1
  MinMax : MinMax  Inputs=4
  MinMax1 : MinMax  Inputs=2
  MinMax2 : MinMax  Inputs=2
  MinMax4 : MinMax  Inputs=2
  ROOut1 : RelationalOperator  Operator===  OutDataTypeStr=boolean  RndMeth=Simplest
  ROOut2 : RelationalOperator  Operator===  OutDataTypeStr=boolean  RndMeth=Simplest
  ROOut4 : RelationalOperator  Operator===  OutDataTypeStr=boolean  RndMeth=Simplest
  Out1 : Outport
  wires:
  Data Type Conversion3/1 -> MinMax4/1
  Data Type Conversion1/1 -> MinMax2/1
  Data Type Conversion/1 -> MinMax1/1
  MinMax1/1 -> Memory1/1, MinMax/1
  ROOut4/1 -> Data Type Conversion3/1
  MinMax2/1 -> Memory2/1, MinMax/2
  ROOut1/1 -> Data Type Conversion/1
  Memory2/1 -> MinMax2/2
  Memory4/1 -> MinMax4/2
  ROOut2/1 -> Data Type Conversion1/1
  MinMax4/1 -> Memory4/1, MinMax/4
  Memory1/1 -> MinMax1/2
  [out4] -> ROOut4/2
  In4/1 -> ROOut4/1
  [out2] -> ROOut2/2
  In1/1 -> ROOut1/1
  In2/1 -> ROOut2/1
  [out1] -> ROOut1/2
  MinMax/1 -> Out1/1
  Constant3/1 -> MinMax/3

== system c00019M_harness/Eval171 ==
  In1 : Inport
  In2 : Inport  Port=2
  In4 : Inport  Port=3
  Constant3 : Constant
  Data Type Conversion : DataTypeConversion
  Data Type Conversion1 : DataTypeConversion
  Data Type Conversion3 : DataTypeConversion
  Memory1 : Memory  InitialCondition=1
  Memory2 : Memory  InitialCondition=1
  Memory4 : Memory  InitialCondition=1
  MinMax : MinMax  Inputs=4
  MinMax1 : MinMax  Inputs=2
  MinMax2 : MinMax  Inputs=2
  MinMax4 : MinMax  Inputs=2
  ROOut1 : RelationalOperator  Operator===  OutDataTypeStr=boolean  RndMeth=Simplest
  ROOut2 : RelationalOperator  Operator===  OutDataTypeStr=boolean  RndMeth=Simplest
  ROOut4 : RelationalOperator  Operator===  OutDataTypeStr=boolean  RndMeth=Simplest
  Out1 : Outport
  wires:
  Data Type Conversion3/1 -> MinMax4/1
  Data Type Conversion1/1 -> MinMax2/1
  Data Type Conversion/1 -> MinMax1/1
  MinMax1/1 -> Memory1/1, MinMax/1
  ROOut4/1 -> Data Type Conversion3/1
  MinMax2/1 -> Memory2/1, MinMax/2
  ROOut1/1 -> Data Type Conversion/1
  Memory2/1 -> MinMax2/2
  Memory4/1 -> MinMax4/2
  ROOut2/1 -> Data Type Conversion1/1
  MinMax4/1 -> Memory4/1, MinMax/4
  Memory1/1 -> MinMax1/2
  [out4] -> ROOut4/2
  In4/1 -> ROOut4/1
  [out2] -> ROOut2/2
  In1/1 -> ROOut1/1
  In2/1 -> ROOut2/1
  [out1] -> ROOut1/2
  MinMax/1 -> Out1/1
  Constant3/1 -> MinMax/3

== system c00019M_harness/Eval173 ==
  In1 : Inport
  In2 : Inport  Port=2
  In4 : Inport  Port=3
  Constant3 : Constant
  Data Type Conversion : DataTypeConversion
  Data Type Conversion1 : DataTypeConversion
  Data Type Conversion3 : DataTypeConversion
  Memory1 : Memory  InitialCondition=1
  Memory2 : Memory  InitialCondition=1
  Memory4 : Memory  InitialCondition=1
  MinMax : MinMax  Inputs=4
  MinMax1 : MinMax  Inputs=2
  MinMax2 : MinMax  Inputs=2
  MinMax4 : MinMax  Inputs=2
  ROOut1 : RelationalOperator  Operator===  OutDataTypeStr=boolean  RndMeth=Simplest
  ROOut2 : RelationalOperator  Operator===  OutDataTypeStr=boolean  RndMeth=Simplest
  ROOut4 : RelationalOperator  Operator===  OutDataTypeStr=boolean  RndMeth=Simplest
  Out1 : Outport
  wires:
  Data Type Conversion3/1 -> MinMax4/1
  Data Type Conversion1/1 -> MinMax2/1
  Data Type Conversion/1 -> MinMax1/1
  MinMax1/1 -> Memory1/1, MinMax/1
  ROOut4/1 -> Data Type Conversion3/1
  MinMax2/1 -> Memory2/1, MinMax/2
  ROOut1/1 -> Data Type Conversion/1
  Memory2/1 -> MinMax2/2
  Memory4/1 -> MinMax4/2
  ROOut2/1 -> Data Type Conversion1/1
  MinMax4/1 -> Memory4/1, MinMax/4
  Memory1/1 -> MinMax1/2
  [out4] -> ROOut4/2
  In4/1 -> ROOut4/1
  [out2] -> ROOut2/2
  In1/1 -> ROOut1/1
  In2/1 -> ROOut2/1
  [out1] -> ROOut1/2
  MinMax/1 -> Out1/1
  Constant3/1 -> MinMax/3

== system c00019M_harness/Eval18 ==
  In1 : Inport
  In2 : Inport  Port=2
  In4 : Inport  Port=3
  Constant3 : Constant
  Data Type Conversion : DataTypeConversion
  Data Type Conversion1 : DataTypeConversion
  Data Type Conversion3 : DataTypeConversion
  Memory1 : Memory  InitialCondition=1
  Memory2 : Memory  InitialCondition=1
  Memory4 : Memory  InitialCondition=1
  MinMax : MinMax  Inputs=4
  MinMax1 : MinMax  Inputs=2
  MinMax2 : MinMax  Inputs=2
  MinMax4 : MinMax  Inputs=2
  ROOut1 : RelationalOperator  Operator===  OutDataTypeStr=boolean  RndMeth=Simplest
  ROOut2 : RelationalOperator  Operator===  OutDataTypeStr=boolean  RndMeth=Simplest
  ROOut4 : RelationalOperator  Operator===  OutDataTypeStr=boolean  RndMeth=Simplest
  Out1 : Outport
  wires:
  Data Type Conversion3/1 -> MinMax4/1
  Data Type Conversion1/1 -> MinMax2/1
  Data Type Conversion/1 -> MinMax1/1
  MinMax1/1 -> Memory1/1, MinMax/1
  ROOut4/1 -> Data Type Conversion3/1
  MinMax2/1 -> Memory2/1, MinMax/2
  ROOut1/1 -> Data Type Conversion/1
  Memory2/1 -> MinMax2/2
  Memory4/1 -> MinMax4/2
  ROOut2/1 -> Data Type Conversion1/1
  MinMax4/1 -> Memory4/1, MinMax/4
  Memory1/1 -> MinMax1/2
  [out4] -> ROOut4/2
  In4/1 -> ROOut4/1
  [out2] -> ROOut2/2
  In1/1 -> ROOut1/1
  In2/1 -> ROOut2/1
  [out1] -> ROOut1/2
  MinMax/1 -> Out1/1
  Constant3/1 -> MinMax/3

== system c00019M_harness/Eval19 ==
  In1 : Inport
  In2 : Inport  Port=2
  In4 : Inport  Port=3
  Constant3 : Constant
  Data Type Conversion : DataTypeConversion
  Data Type Conversion1 : DataTypeConversion
  Data Type Conversion3 : DataTypeConversion
  Memory1 : Memory  InitialCondition=1
  Memory2 : Memory  InitialCondition=1
  Memory4 : Memory  InitialCondition=1
  MinMax : MinMax  Inputs=4
  MinMax1 : MinMax  Inputs=2
  MinMax2 : MinMax  Inputs=2
  MinMax4 : MinMax  Inputs=2
  ROOut1 : RelationalOperator  Operator===  OutDataTypeStr=boolean  RndMeth=Simplest
  ROOut2 : RelationalOperator  Operator===  OutDataTypeStr=boolean  RndMeth=Simplest
  ROOut4 : RelationalOperator  Operator===  OutDataTypeStr=boolean  RndMeth=Simplest
  Out1 : Outport
  wires:
  Data Type Conversion3/1 -> MinMax4/1
  Data Type Conversion1/1 -> MinMax2/1
  Data Type Conversion/1 -> MinMax1/1
  MinMax1/1 -> Memory1/1, MinMax/1
  ROOut4/1 -> Data Type Conversion3/1
  MinMax2/1 -> Memory2/1, MinMax/2
  ROOut1/1 -> Data Type Conversion/1
  Memory2/1 -> MinMax2/2
  Memory4/1 -> MinMax4/2
  ROOut2/1 -> Data Type Conversion1/1
  MinMax4/1 -> Memory4/1, MinMax/4
  Memory1/1 -> MinMax1/2
  [out4] -> ROOut4/2
  In4/1 -> ROOut4/1
  [out2] -> ROOut2/2
  In1/1 -> ROOut1/1
  In2/1 -> ROOut2/1
  [out1] -> ROOut1/2
  MinMax/1 -> Out1/1
  Constant3/1 -> MinMax/3

== system c00019M_harness/Eval2 ==
  In1 : Inport
  In2 : Inport  Port=2
  In4 : Inport  Port=3
  Constant3 : Constant
  Data Type Conversion : DataTypeConversion
  Data Type Conversion1 : DataTypeConversion
  Data Type Conversion3 : DataTypeConversion
  Memory1 : Memory  InitialCondition=1
  Memory2 : Memory  InitialCondition=1
  Memory4 : Memory  InitialCondition=1
  MinMax : MinMax  Inputs=4
  MinMax1 : MinMax  Inputs=2
  MinMax2 : MinMax  Inputs=2
  MinMax4 : MinMax  Inputs=2
  ROOut1 : RelationalOperator  Operator===  OutDataTypeStr=boolean  RndMeth=Simplest
  ROOut2 : RelationalOperator  Operator===  OutDataTypeStr=boolean  RndMeth=Simplest
  ROOut4 : RelationalOperator  Operator===  OutDataTypeStr=boolean  RndMeth=Simplest
  Out1 : Outport
  wires:
  Data Type Conversion3/1 -> MinMax4/1
  Data Type Conversion1/1 -> MinMax2/1
  Data Type Conversion/1 -> MinMax1/1
  MinMax1/1 -> Memory1/1, MinMax/1
  ROOut4/1 -> Data Type Conversion3/1
  MinMax2/1 -> Memory2/1, MinMax/2
  ROOut1/1 -> Data Type Conversion/1
  Memory2/1 -> MinMax2/2
  Memory4/1 -> MinMax4/2
  ROOut2/1 -> Data Type Conversion1/1
  MinMax4/1 -> Memory4/1, MinMax/4
  Memory1/1 -> MinMax1/2
  [out4] -> ROOut4/2
  In4/1 -> ROOut4/1
  [out2] -> ROOut2/2
  In1/1 -> ROOut1/1
  In2/1 -> ROOut2/1
  [out1] -> ROOut1/2
  MinMax/1 -> Out1/1
  Constant3/1 -> MinMax/3

== system c00019M_harness/Eval21 ==
  In1 : Inport
  In2 : Inport  Port=2
  In4 : Inport  Port=3
  Constant3 : Constant
  Data Type Conversion : DataTypeConversion
  Data Type Conversion1 : DataTypeConversion
  Data Type Conversion3 : DataTypeConversion
  Memory1 : Memory  InitialCondition=1
  Memory2 : Memory  InitialCondition=1
  Memory4 : Memory  InitialCondition=1
  MinMax : MinMax  Inputs=4
  MinMax1 : MinMax  Inputs=2
  MinMax2 : MinMax  Inputs=2
  MinMax4 : MinMax  Inputs=2
  ROOut1 : RelationalOperator  Operator===  OutDataTypeStr=boolean  RndMeth=Simplest
  ROOut2 : RelationalOperator  Operator===  OutDataTypeStr=boolean  RndMeth=Simplest
  ROOut4 : RelationalOperator  Operator===  OutDataTypeStr=boolean  RndMeth=Simplest
  Out1 : Outport
  wires:
  Data Type Conversion3/1 -> MinMax4/1
  Data Type Conversion1/1 -> MinMax2/1
  Data Type Conversion/1 -> MinMax1/1
  MinMax1/1 -> Memory1/1, MinMax/1
  ROOut4/1 -> Data Type Conversion3/1
  MinMax2/1 -> Memory2/1, MinMax/2
  ROOut1/1 -> Data Type Conversion/1
  Memory2/1 -> MinMax2/2
  Memory4/1 -> MinMax4/2
  ROOut2/1 -> Data Type Conversion1/1
  MinMax4/1 -> Memory4/1, MinMax/4
  Memory1/1 -> MinMax1/2
  [out4] -> ROOut4/2
  In4/1 -> ROOut4/1
  [out2] -> ROOut2/2
  In1/1 -> ROOut1/1
  In2/1 -> ROOut2/1
  [out1] -> ROOut1/2
  MinMax/1 -> Out1/1
  Constant3/1 -> MinMax/3

== system c00019M_harness/Eval22 ==
  In1 : Inport
  In2 : Inport  Port=2
  In4 : Inport  Port=3
  Constant3 : Constant
  Data Type Conversion : DataTypeConversion
  Data Type Conversion1 : DataTypeConversion
  Data Type Conversion3 : DataTypeConversion
  Memory1 : Memory  InitialCondition=1
  Memory2 : Memory  InitialCondition=1
  Memory4 : Memory  InitialCondition=1
  MinMax : MinMax  Inputs=4
  MinMax1 : MinMax  Inputs=2
  MinMax2 : MinMax  Inputs=2
  MinMax4 : MinMax  Inputs=2
  ROOut1 : RelationalOperator  Operator===  OutDataTypeStr=boolean  RndMeth=Simplest
  ROOut2 : RelationalOperator  Operator===  OutDataTypeStr=boolean  RndMeth=Simplest
  ROOut4 : RelationalOperator  Operator===  OutDataTypeStr=boolean  RndMeth=Simplest
  Out1 : Outport
  wires:
  Data Type Conversion3/1 -> MinMax4/1
  Data Type Conversion1/1 -> MinMax2/1
  Data Type Conversion/1 -> MinMax1/1
  MinMax1/1 -> Memory1/1, MinMax/1
  ROOut4/1 -> Data Type Conversion3/1
  MinMax2/1 -> Memory2/1, MinMax/2
  ROOut1/1 -> Data Type Conversion/1
  Memory2/1 -> MinMax2/2
  Memory4/1 -> MinMax4/2
  ROOut2/1 -> Data Type Conversion1/1
  MinMax4/1 -> Memory4/1, MinMax/4
  Memory1/1 -> MinMax1/2
  [out4] -> ROOut4/2
  In4/1 -> ROOut4/1
  [out2] -> ROOut2/2
  In1/1 -> ROOut1/1
  In2/1 -> ROOut2/1
  [out1] -> ROOut1/2
  MinMax/1 -> Out1/1
  Constant3/1 -> MinMax/3

== system c00019M_harness/Eval23 ==
  In1 : Inport
  In2 : Inport  Port=2
  In4 : Inport  Port=3
  Constant3 : Constant
  Data Type Conversion : DataTypeConversion
  Data Type Conversion1 : DataTypeConversion
  Data Type Conversion3 : DataTypeConversion
  Memory1 : Memory  InitialCondition=1
  Memory2 : Memory  InitialCondition=1
  Memory4 : Memory  InitialCondition=1
  MinMax : MinMax  Inputs=4
  MinMax1 : MinMax  Inputs=2
  MinMax2 : MinMax  Inputs=2
  MinMax4 : MinMax  Inputs=2
  ROOut1 : RelationalOperator  Operator===  OutDataTypeStr=boolean  RndMeth=Simplest
  ROOut2 : RelationalOperator  Operator===  OutDataTypeStr=boolean  RndMeth=Simplest
  ROOut4 : RelationalOperator  Operator===  OutDataTypeStr=boolean  RndMeth=Simplest
  Out1 : Outport
  wires:
  Data Type Conversion3/1 -> MinMax4/1
  Data Type Conversion1/1 -> MinMax2/1
  Data Type Conversion/1 -> MinMax1/1
  MinMax1/1 -> Memory1/1, MinMax/1
  ROOut4/1 -> Data Type Conversion3/1
  MinMax2/1 -> Memory2/1, MinMax/2
  ROOut1/1 -> Data Type Conversion/1
  Memory2/1 -> MinMax2/2
  Memory4/1 -> MinMax4/2
  ROOut2/1 -> Data Type Conversion1/1
  MinMax4/1 -> Memory4/1, MinMax/4
  Memory1/1 -> MinMax1/2
  [out4] -> ROOut4/2
  In4/1 -> ROOut4/1
  [out2] -> ROOut2/2
  In1/1 -> ROOut1/1
  In2/1 -> ROOut2/1
  [out1] -> ROOut1/2
  MinMax/1 -> Out1/1
  Constant3/1 -> MinMax/3

== system c00019M_harness/Eval25 ==
  In1 : Inport
  In2 : Inport  Port=2
  In4 : Inport  Port=3
  Constant3 : Constant
  Data Type Conversion : DataTypeConversion
  Data Type Conversion1 : DataTypeConversion
  Data Type Conversion3 : DataTypeConversion
  Memory1 : Memory  InitialCondition=1
  Memory2 : Memory  InitialCondition=1
  Memory4 : Memory  InitialCondition=1
  MinMax : MinMax  Inputs=4
  MinMax1 : MinMax  Inputs=2
  MinMax2 : MinMax  Inputs=2
  MinMax4 : MinMax  Inputs=2
  ROOut1 : RelationalOperator  Operator===  OutDataTypeStr=boolean  RndMeth=Simplest
  ROOut2 : RelationalOperator  Operator===  OutDataTypeStr=boolean  RndMeth=Simplest
  ROOut4 : RelationalOperator  Operator===  OutDataTypeStr=boolean  RndMeth=Simplest
  Out1 : Outport
  wires:
  Data Type Conversion3/1 -> MinMax4/1
  Data Type Conversion1/1 -> MinMax2/1
  Data Type Conversion/1 -> MinMax1/1
  MinMax1/1 -> Memory1/1, MinMax/1
  ROOut4/1 -> Data Type Conversion3/1
  MinMax2/1 -> Memory2/1, MinMax/2
  ROOut1/1 -> Data Type Conversion/1
  Memory2/1 -> MinMax2/2
  Memory4/1 -> MinMax4/2
  ROOut2/1 -> Data Type Conversion1/1
  MinMax4/1 -> Memory4/1, MinMax/4
  Memory1/1 -> MinMax1/2
  [out4] -> ROOut4/2
  In4/1 -> ROOut4/1
  [out2] -> ROOut2/2
  In1/1 -> ROOut1/1
  In2/1 -> ROOut2/1
  [out1] -> ROOut1/2
  MinMax/1 -> Out1/1
  Constant3/1 -> MinMax/3

== system c00019M_harness/Eval26 ==
  In1 : Inport
  In2 : Inport  Port=2
  In4 : Inport  Port=3
  Constant3 : Constant
  Data Type Conversion : DataTypeConversion
  Data Type Conversion1 : DataTypeConversion
  Data Type Conversion3 : DataTypeConversion
  Memory1 : Memory  InitialCondition=1
  Memory2 : Memory  InitialCondition=1
  Memory4 : Memory  InitialCondition=1
  MinMax : MinMax  Inputs=4
  MinMax1 : MinMax  Inputs=2
  MinMax2 : MinMax  Inputs=2
  MinMax4 : MinMax  Inputs=2
  ROOut1 : RelationalOperator  Operator===  OutDataTypeStr=boolean  RndMeth=Simplest
  ROOut2 : RelationalOperator  Operator===  OutDataTypeStr=boolean  RndMeth=Simplest
  ROOut4 : RelationalOperator  Operator===  OutDataTypeStr=boolean  RndMeth=Simplest
  Out1 : Outport
  wires:
  Data Type Conversion3/1 -> MinMax4/1
  Data Type Conversion1/1 -> MinMax2/1
  Data Type Conversion/1 -> MinMax1/1
  MinMax1/1 -> Memory1/1, MinMax/1
  ROOut4/1 -> Data Type Conversion3/1
  MinMax2/1 -> Memory2/1, MinMax/2
  ROOut1/1 -> Data Type Conversion/1
  Memory2/1 -> MinMax2/2
  Memory4/1 -> MinMax4/2
  ROOut2/1 -> Data Type Conversion1/1
  MinMax4/1 -> Memory4/1, MinMax/4
  Memory1/1 -> MinMax1/2
  [out4] -> ROOut4/2
  In4/1 -> ROOut4/1
  [out2] -> ROOut2/2
  In1/1 -> ROOut1/1
  In2/1 -> ROOut2/1
  [out1] -> ROOut1/2
  MinMax/1 -> Out1/1
  Constant3/1 -> MinMax/3
